simulink model "Heli_2dof"  (R2022a)
settings: Solver=VariableStepAuto  StartTime=0.0  StopTime=30  RelTol=1e-3
undefined symbols (not defined in the file): sigbuilder_block
settings Model: Creator=dmonge  LastModifiedBy=dmonge

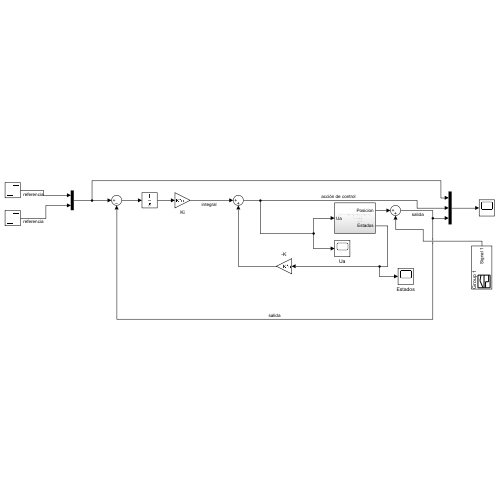
[thumbnail: Simulink's stored preview of the top-level diagram]
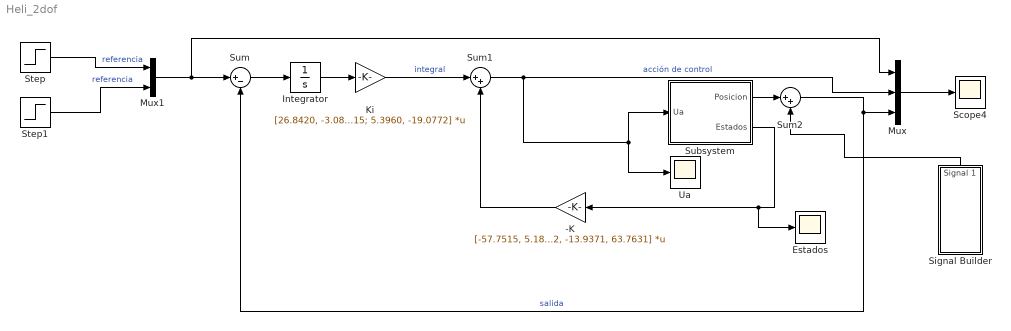
== system Heli_2dof ==
  -K : Gain  Gain=[-57.7515, 5.1894, -28.8388, 1.9559; -7.7602, 62.0422, -13.9371, 63.7631]  Multiplication=Matrix(K*u)
  Estados : Scope
  Integrator : Integrator
  Ki : Gain  Gain=[26.8420, -3.0815; 5.3960, -19.0772]  Multiplication=Matrix(K*u)
  Mux : Mux  Inputs=3
  Mux1 : Mux  Inputs=2
  Scope4 : Scope
  Signal Builder : Subsystem  Tag=STV Subsys  LoadFcn=sigbuilder_block('load');  StartFcn=sigbuilder_block('start');  StopFcn=sigbuilder_block('stop');  ClipboardFcn=sigbuilder_block('clipboard');  mask(Sigbuilder block){tuvar=[0:10]}
      mask help: Simulink:masks:SigbuilderBlock_MD
      mask init:
      | if ~strcmp(get_param(bdroot(gcbh),'SimulationStatus'),'stopped') tuvar = sigbuilder_block('maskInit'); end
      settings: CopyFcn=sigbuilder_block('copy');  DeleteFcn=sigbuilder_block('delete');  ModelCloseFcn=sigbuilder_block('modelClose');  PreSaveFcn=sigbuilder_block('preSave');  PauseFcn=sigbuilder_block('pause');  ContinueFcn=sigbuilder_block('continue');  NameChangeFcn=sigbuilder_block('namechange');  OpenFcn=sigbuilder_block('open',[334.8 88.8 550.8 400.2 ]);  CloseFcn=sigbuilder_block('close');
      mask Display: plot(0, 0, 100, 100,[2, 2, 32, 32, 2], [68, 8, 8, 68, 68],[32, 2], [38, 38], [32, 19, 2],[53, 60, 44], [32, 17, 17, 2],[16, 16, 31, 31]);txt = getActiveGroup(gcbh);text(2, 100, txt,'verticalAlignment', 'top');
  Step : Step  Time=0  After=0.583  SampleTime=0
  Step1 : Step  Time=0  After=0  SampleTime=0
  Subsystem : Subsystem
  Sum : Sum  Inputs=|+-
  Sum1 : Sum  Inputs=|++
  Sum2 : Sum  Inputs=|++
  Ua : Scope
  wires:
  Integrator/1 -> Ki/1
  Signal Builder/1(Signal 1) -> Sum2/2
  Step1/1 -> Mux1/2  "referencia"
  Mux/1 -> Scope4/1
  Ki/1 -> Sum1/1  "integral"
  Sum/1 -> Integrator/1
  Sum2/1 -> Mux/3, Sum/2  "salida"
  Subsystem/2(Estados) -> Estados/1, -K/1
  Subsystem/1(Posicion) -> Sum2/1
  -K/1 -> Sum1/2
  Step/1 -> Mux1/1  "referencia"
  Mux1/1 -> Mux/1, Sum/1
  Sum1/1 -> Ua/1, Subsystem/1(Ua), Mux/2  "acción de control"

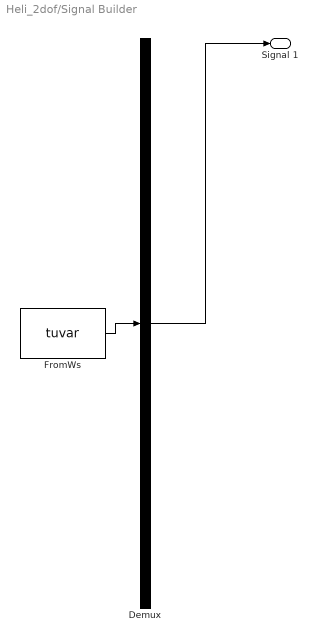
== system Heli_2dof/Signal Builder ==
  Demux : Demux  Tag=STV Demux  Outputs=1
      settings: DisplayOption=none
  FromWs : FromWorkspace  Tag=STV FromWs  VariableName=tuvar
      SigBuilderData=|
      | common.afterFinalStr = 'Extrapolate'
      | common.sampleTime = 0
      | dataSet.timeRange = [0 30]
      | dataSet.name = 'Group 1'
      | sbobj.Groups.Name = 'Group 1'
      | sbobj.Groups.Signals.Name = 'Signal 1'
      | sbobj.Groups.Signals.XData = [0 15 16 19 20 30]
      | sbobj.Groups.Signals.YData = [0 0 0.05 0.05 0 0]
      | sbobj.Groups.TimeRange = [0 30]
  Signal 1 : Outport  Tag=STV Outport
  wires:
  Demux/1 -> Signal 1/1
  FromWs/1 -> Demux/1

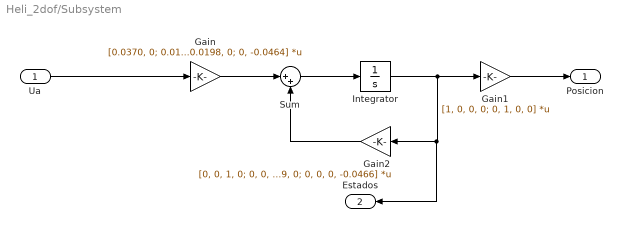
== system Heli_2dof/Subsystem ==
  Ua : Inport
  Gain : Gain  Gain=[0.0370, 0; 0.0131, 0; 0.0198, 0; 0, -0.0464]  Multiplication=Matrix(K*u)
  Gain1 : Gain  Gain=[1, 0, 0, 0; 0, 1, 0, 0]  Multiplication=Matrix(K*u)
  Gain2 : Gain  Gain=[0, 0, 1, 0; 0, 0, 0, 1; -1.0930, 0, -0.6029, 0; 0, 0, 0, -0.0466]  Multiplication=Matrix(K*u)
  Integrator : Integrator
  Sum : Sum  Inputs=|++
  Posicion : Outport
  Estados : Outport  Port=2
  wires:
  Gain/1 -> Sum/1
  Integrator/1 -> Estados/1, Gain2/1, Gain1/1
  Sum/1 -> Integrator/1
  Gain2/1 -> Sum/2
  Gain1/1 -> Posicion/1
  Ua/1 -> Gain/1
